simulink model "TV_2017"  (R2016a)
settings: Solver=FixedStepAuto  StartTime=0.0  StopTime=inf  FixedStep=0.001  RelTol=1e-3
PreLoadFcn:
  | TV_2017_parameters
values from neighbouring files (symbols this model uses):
  battery_voltage = single(530)    [HIL_parameters.m]    (also in HIL_parameters_2018.m; TV_2017_parameters.m; TV_2017_parameters_VD.m)
  car_params = Simulink_Car_params    [HIL_parameters.m]    (also in HIL_parameters_2018.m; TV_2017_parameters.m; TV_2017_parameters_VD.m)
  i_Diff = 16    [HIL_parameters.m]    (also in HIL_parameters_2018.m; TV_2017_parameters.m)
  Kp = 1    [HIL_parameters.m]    (also in HIL_parameters_2018.m; TV_2017_parameters.m; TV_2017_parameters_VD.m)
  motor_data = struct    [HIL_parameters.m]    (also in HIL_parameters_2018.m; TV_2017_parameters.m)
  powerLimitControl = Simulink_el    [HIL_parameters.m]    (also in HIL_parameters_2018.m; TV_2017_parameters.m; TV_2017_parameters_VD.m)
  settings = Simulink_Settings    [HIL_parameters.m]    (also in HIL_parameters_2018.m; TV_2017_parameters.m; TV_2017_parameters_VD.m)
  SpdC_BCC = 0    [HIL_parameters.m]    (also in HIL_parameters_2018.m; TV_2017_parameters.m; TV_2017_parameters_VD.m)
  Speed_Neg_sat = -21    [HIL_parameters.m]    (also in HIL_parameters_2018.m; TV_2017_parameters.m; TV_2017_parameters_VD.m)
  Speed_Pos_sat = 21    [HIL_parameters.m]    (also in HIL_parameters_2018.m; TV_2017_parameters.m; TV_2017_parameters_VD.m)
  SteeringAngleFL = [-23.80 -22.65 -21.50 -20.34 -19.18 -18.03 -16.86 -15.70 -14.53 -13.35 -12.18 -10.99 -9.80 -8.61 -7.40 -6.19 -4.97 -3.75 -2.51 -1.26 0 1.27 2.56 3.85 5.17 6.50 7.84 9.21 10.59 12.00 13.42 14.88 16.36 17.87 19.41 20.99 22.61 24.26 25.97 27.73 29.54]    [CarSetupAnalysis2018.m]    (also in HIL_parameters_2018.m; TV_2017_parameters.m; TV_2017_parameters_VD.m = [-24.129 -22.950 -21.772 -20.593 -19.413 -18.232 -17.050 -15)
  SteeringAngleFR = [-29.54 -27.73 -25.97 -24.26 -22.61 -20.99 -19.41 -17.87 -16.36 -14.88 -13.42 -12.00 -10.59 -9.21 -7.84 -6.50 -5.17 -3.85 -2.56 -1.27 0 1.26 2.51 3.75 4.97 6.19 7.40 8.61 9.80 10.99 12.18 13.35 14.53 15.70 16.86 18.03 19.18 20.34 21.50 22.65 23.80]    [CarSetupAnalysis2018.m]    (also in HIL_parameters_2018.m; TV_2017_parameters.m; TV_2017_parameters_VD.m = [-29.3050 -27.5340 -25.8140 -24.1410 -22.5110 -20.9180 -19.3)
  SteeringWhAngle = [-105 -99.75 -94.5 -89.25 -84 -78.75 -73.5 -68.25 -63 -57.75 -52.5 -47.25 -42 -36.75 -31.5 -26.25 -21.0 -15.75 -10.5 -5.25 0.0 5.25 10.50 15.75 21.00 26.25 31.50 36.75 42.00 47.25 52.50 57.75  63.00 68.25 73.50 78.75 84.00 89.25 94.50 99.75 105.00]    [TV_2017_parameters_VD.m]
  Tn_n = 0    [HIL_parameters.m]    (also in HIL_parameters_2018.m; TV_2017_parameters.m; TV_2017_parameters_VD.m)
  tractionControl = Simulink_tc    [HIL_parameters.m]    (also in HIL_parameters_2018.m; IterativeTractionControlTuning.m; TV_2017_parameters.m; TV_2017_parameters_VD.m)
  yawMomentGenerator = struct    [HIL_parameters.m]    (also in HIL_parameters_2018.m = Simulink_yawRate2; TV_2017_parameters.m = Simulink_yawRate2)
  yawRateControl = Simulink_yawRate    [HIL_parameters.m]    (also in HIL_parameters_2018.m; TV_2017_parameters.m; TV_2017_parameters_VD.m)
undefined symbols (not defined in the file or in its folder): DiscIntNeverNeededParam, magnitude, speedEstimation, TC_Decr_Gas, TC_Derivative, TC_Incr_Gas, TC_On, TC_Relay_Off, TC_Relay_On
libraries: CarMaker4SL x350, simulink_extras x63, simulink x37, dspfdesign x2
(part 5 of 14)

== system TV_2017/CarMaker/Estimations/createStateBus ==
  mean_wheel_angle : Inport
  mean_wheel_speed : Inport  Port=2
  Fx : Inport  Port=3
  sensors : Inport  Port=4
  Fz_est : Inport  Port=5
  whl_speed_cog : Inport  Port=6
  SR : Inport  Port=7
  frictionCoefficient : Inport  Port=8
  SA : Inport  Port=9
  v_x : Inport  Port=10
  v_y : Inport  Port=11
  slip : Inport  Port=12
  Bus Creator1 : BusCreator  Inputs=52  OutDataTypeStr=Bus: States  NonVirtualBus=on
      settings: InheritFromInputs=off
  Bus Selector{,2..6} (6 alike) : BusSelector  OutputSignals=FL,FR,RL,RR
  Bus Selector1 : BusSelector  OutputSignals=Input_throttle,Input_brake,KERS_pos,yawRate,yawRate_der,ax,ay,RPM_FL,RPM_FR,RPM_RL,RPM_RR,power,DC_voltage,AMK_motor_temp_FL,AMK_motor_temp_FR,AMK_motor_temp_RL,AMK_motor_temp_RR,AMK_inverter_temp_FL,AMK_inverter_temp_FR,AMK_inverter_temp_RL,AMK_inverter_temp_RR,steering_wheel_angle,steering_wheel_speed
  states : Outport
  wires:
  sensors/1 -> Bus Selector1/1
  Fz_est/1 -> Bus Selector/1
  whl_speed_cog/1 -> Bus Selector2/1
  Fx/1 -> Bus Selector3/1
  SR/1 -> Bus Selector4/1
  Bus Selector1/9 -> Bus Creator1/9  "<RPM_FR>"
  Bus Selector1/8 -> Bus Creator1/8  "<RPM_FL>"
  Bus Selector1/10 -> Bus Creator1/10  "<RPM_RL>"
  Bus Selector1/7 -> Bus Creator1/7  "<ay>"
  Bus Selector1/11 -> Bus Creator1/11  "<RPM_RR>"
  Bus Selector1/6 -> Bus Creator1/6  "<ax>"
  Bus Selector1/12 -> Bus Creator1/12  "<power>"
  Bus Selector1/5 -> Bus Creator1/5  "<yawRate_der>"
  Bus Selector1/13 -> Bus Creator1/13  "<DC_voltage>"
  Bus Selector1/4 -> Bus Creator1/4  "<yawRate>"
  Bus Selector1/3 -> Bus Creator1/3  "<KERS_pos>"
  Bus Selector1/2 -> Bus Creator1/2  "<Input_brake>"
  Bus Selector1/1 -> Bus Creator1/1  "<Input_throttle>"
  mean_wheel_angle/1 -> Bus Creator1/24
  mean_wheel_speed/1 -> Bus Creator1/25
  v_x/1 -> Bus Creator1/26
  v_y/1 -> Bus Creator1/27
  Bus Selector/1 -> Bus Creator1/32  "<FL>"
  Bus Selector/2 -> Bus Creator1/33  "<FR>"
  Bus Selector/3 -> Bus Creator1/34  "<RL>"
  Bus Selector/4 -> Bus Creator1/35  "<RR>"
  Bus Selector2/1 -> Bus Creator1/36  "<FL>"
  Bus Selector2/2 -> Bus Creator1/37  "<FR>"
  Bus Selector2/3 -> Bus Creator1/38  "<RL>"
  Bus Selector2/4 -> Bus Creator1/39  "<RR>"
  Bus Selector4/1 -> Bus Creator1/40  "<FL>"
  Bus Selector4/2 -> Bus Creator1/41  "<FR>"
  Bus Selector4/3 -> Bus Creator1/42  "<RL>"
  Bus Selector4/4 -> Bus Creator1/43  "<RR>"
  Bus Selector3/1 -> Bus Creator1/28  "<FL>"
  Bus Selector3/2 -> Bus Creator1/29  "<FR>"
  Bus Selector3/3 -> Bus Creator1/30  "<RL>"
  Bus Selector3/4 -> Bus Creator1/31  "<RR>"
  frictionCoefficient/1 -> Bus Creator1/52
  Bus Selector1/14 -> Bus Creator1/14  "<AMK_motor_temp_FL>"
  Bus Selector1/15 -> Bus Creator1/15  "<AMK_motor_temp_FR>"
  Bus Selector1/16 -> Bus Creator1/16  "<AMK_motor_temp_RL>"
  Bus Selector1/17 -> Bus Creator1/17  "<AMK_motor_temp_RR>"
  Bus Selector1/18 -> Bus Creator1/18  "<AMK_inverter_temp_FL>"
  Bus Selector1/19 -> Bus Creator1/19  "<AMK_inverter_temp_FR>"
  Bus Selector1/20 -> Bus Creator1/20  "<AMK_inverter_temp_RL>"
  Bus Selector1/21 -> Bus Creator1/21  "<AMK_inverter_temp_RR>"
  SA/1 -> Bus Selector5/1
  Bus Selector5/1 -> Bus Creator1/44  "<FL>"
  Bus Selector5/2 -> Bus Creator1/45  "<FR>"
  Bus Selector5/3 -> Bus Creator1/46  "<RL>"
  Bus Selector5/4 -> Bus Creator1/47  "<RR>"
  Bus Creator1/1 -> states/1
  Bus Selector1/22 -> Bus Creator1/22  "<steering_wheel_angle>"
  Bus Selector1/23 -> Bus Creator1/23  "<steering_wheel_speed>"
  slip/1 -> Bus Selector6/1
  Bus Selector6/1 -> Bus Creator1/48  "<FL>"
  Bus Selector6/2 -> Bus Creator1/49  "<FR>"
  Bus Selector6/3 -> Bus Creator1/50  "<RL>"
  Bus Selector6/4 -> Bus Creator1/51  "<RR>"

== system TV_2017/CarMaker/Estimations/friction_estimation ==
  Fx : Inport
  SR : Inport  Port=2
  Fz : Inport  Port=3
  estimateFrictionCoefficient : MATLAB Function  TreatAsAtomicUnit=on
  mu : Outport
  mu_estimate : Outport  Port=2
  mu_individual : Outport  Port=3
  normLongTireForce : Outport  Port=4
  wires:
  Fx/1 -> estimateFrictionCoefficient/1(Fx)
  Fz/1 -> estimateFrictionCoefficient/2(Fz)
  SR/1 -> estimateFrictionCoefficient/3(SR)
  estimateFrictionCoefficient/1(mu) -> mu/1
  estimateFrictionCoefficient/3(normLongTireForce) -> normLongTireForce/1
  estimateFrictionCoefficient/2(mu_estimate) -> mu_estimate/1

== system TV_2017/CarMaker/Estimations/selectVelocity ==
  v_est_x : Inport
  sensors : Inport  Port=2
  Bus Selector : BusSelector  OutputSignals=V_x_INS,V_x_optical
  Bus Selector1 : BusSelector  OutputSignals=V_y_INS,V_y_optical
  Constant1 : Constant  Value=settings.select_velocity_vx
  Constant2 : Constant  Value=settings.select_velocity_vy
  Index Vector : MultiPortSwitch
  Index Vector1 : MultiPortSwitch  DataPortOrder=Specify indices  Inputs=2  DataPortIndices={2,3}
  v_x : Outport
  v_y : Outport  Port=2
  wires:
  Constant1/1 -> Index Vector/1
  v_est_x/1 -> Index Vector/2
  sensors/1 -> Bus Selector1/1, Bus Selector/1
  Bus Selector/1 -> Index Vector/3  "<V_x_INS>"
  Bus Selector/2 -> Index Vector/4  "<V_x_optical>"
  Index Vector/1 -> v_x/1
  Constant2/1 -> Index Vector1/1
  Bus Selector1/1 -> Index Vector1/2  "<V_y_INS>"
  Bus Selector1/2 -> Index Vector1/3  "<V_y_optical>"
  Index Vector1/1 -> v_y/1

== system TV_2017/CarMaker/IPG Vehicle3/Brake ==
  note: When replacing the entire braking system,
      | be sure to add '-disablebrake' to the command line arguments
      | in the CarMaker Model Configuration block.
  note: <Your model here>
  Sync_In : Inport
  Brake.IF.In : Inport  Port=2
  VhclCtrl.Brake : Inport  Port=3
  Brake : S-Function  FunctionName=CM_Sfun  Parameters='Brake'  SFunctionDeploymentMode=off  EnableBusSupport=off
  BrakeUpd : S-Function  FunctionName=CM_Sfun  Parameters='BrakeUpd'  SFunctionDeploymentMode=off  EnableBusSupport=off
  BusCreator1 : BusCreator  Inputs=16
  CreateBus Vhcl.Wheel.PT : Subsystem
  Demux : Demux  Outputs=16
  Sync_Out : Outport
  Vhcl.Wheel.PT : Outport  Port=2
  wires:
  Demux/16 -> BusCreator1/16  "Brake IF Trq_DriveSrc_trg d3"
  Demux/15 -> BusCreator1/15  "Brake IF Trq_DriveSrc_trg d2"
  Demux/14 -> BusCreator1/14  "Brake IF Trq_DriveSrc_trg d1"
  Demux/13 -> BusCreator1/13  "Brake IF Trq_DriveSrc_trg d0"
  Demux/12 -> BusCreator1/12  "Brake IF Trq_Reg_trg RR"
  Demux/11 -> BusCreator1/11  "Brake IF Trq_Reg_trg RL"
  Demux/10 -> BusCreator1/10  "Brake IF Trq_Reg_trg FR"
  Demux/9 -> BusCreator1/9  "Brake IF Trq_Reg_trg FL"
  Demux/8 -> BusCreator1/8  "Brake IF Trq_PB RR"
  Demux/7 -> BusCreator1/7  "Brake IF Trq_PB RL"
  Demux/6 -> BusCreator1/6  "Brake IF Trq_PB FR"
  Demux/5 -> BusCreator1/5  "Brake IF Trq_PB FL"
  Demux/4 -> BusCreator1/4  "Brake IF Trq_WB RR"
  Demux/3 -> BusCreator1/3  "Brake IF Trq_WB RL"
  Demux/2 -> BusCreator1/2  "Brake IF Trq_WB FR"
  Demux/1 -> BusCreator1/1  "Brake IF Trq_WB FL"
  Brake/2 -> Demux/1
  BusCreator1/1 -> BrakeUpd/2
  BrakeUpd/1 -> Sync_Out/1
  Brake/1 -> BrakeUpd/1  "Sync"
  Brake.IF.In/1 -> Brake/2
  VhclCtrl.Brake/1 -> Brake/3
  Sync_In/1 -> Brake/1
  BrakeUpd/2 -> CreateBus Vhcl.Wheel.PT/1(In)
  CreateBus Vhcl.Wheel.PT/1(Out) -> Vhcl.Wheel.PT/1

== system TV_2017/CarMaker/IPG Vehicle3/CarAndTrailer ==
  Sync_In : Inport
  VhclCtrl.Steering : Inport  Port=2
  Vhcl.Wheel.In : Inport  Port=3
  Vhcl.Misc : Inport  Port=4
  CarAndTrailerUpd : Subsystem
  Forces : Subsystem
  Ground : Ground
  Kinematics : Subsystem
  Kinetics : Subsystem
  Steering : Subsystem
  Terminator : Terminator
  Terminator1 : Terminator
  Trailer : Subsystem
  Sync_Out : Outport
  Brake.IF.In : Outport  Port=2
  wires:
  Trailer/9(Car.Hitch.FrcTrq) -> CarAndTrailerUpd/9(Car.Hitch.FrcTrq)
  Trailer/8(Vhcl.Wheel.RR) -> CarAndTrailerUpd/8(Vhcl.Wheel.RR)
  Trailer/7(Vhcl.Wheel.RL) -> CarAndTrailerUpd/7(Vhcl.Wheel.RL)
  Trailer/6(Vhcl.Wheel.FR) -> CarAndTrailerUpd/6(Vhcl.Wheel.FR)
  Trailer/5(Vhcl.Wheel.FL) -> CarAndTrailerUpd/5(Vhcl.Wheel.FL)
  Trailer/4(Vhcl.PoI) -> CarAndTrailerUpd/4(Vhcl.PoI)
  Trailer/3(Vhcl.Motion) -> CarAndTrailerUpd/3(Vhcl.Motion)
  Trailer/2(Vhcl.Steering) -> CarAndTrailerUpd/2(Vhcl.Steering)
  Trailer/1(Sync_Out) -> CarAndTrailerUpd/1(Sync_In)
  CarAndTrailerUpd/2(Brake.IF.In) -> Brake.IF.In/1
  CarAndTrailerUpd/1(Sync_Out) -> Sync_Out/1
  Vhcl.Misc/1 -> Terminator1/1
  Vhcl.Wheel.In/1 -> Terminator/1
  Kinetics/6(WheelCarrier.Misc) -> Trailer/6(WheelCarrier.Misc)
  Kinetics/5(Car.Trq_T2W) -> Trailer/5(Car.Trq_T2W)
  Steering/2(Steer.IF) -> Kinematics/2(Steer.IF)
  Kinetics/4(Car.Fr1) -> Trailer/4(Car.Fr1)
  Kinetics/3(Car.Hitch) -> Trailer/3(Car.Hitch)
  Kinetics/2(Trailer.Load) -> Trailer/2(Trailer.Load)
  VhclCtrl.Steering/1 -> Steering/2(VhclCtrl.Steering)
  Sync_In/1 -> Steering/1(Sync_In)
  Steering/1(Sync_Out) -> Kinematics/1(Sync_In)
  Kinetics/1(Sync_Out) -> Trailer/1(Sync_In)
  Ground/1 -> CarAndTrailerUpd/10(Vhcl.Fr1A)
  Forces/11(FStabi) -> Kinetics/11(FStabi)
  Forces/10(FDamp) -> Kinetics/10(FDamp)
  Forces/9(FSpring) -> Kinetics/9(FSpring)
  Forces/8(TireRR_Out) -> Kinetics/8(TireRR.Out)
  Forces/7(TireRL_Out) -> Kinetics/7(TireRL.Out)
  Forces/6(TireFR_Out) -> Kinetics/6(TireFR.Out)
  Forces/5(TireFL_Out) -> Kinetics/5(TireFL.Out)
  Forces/4(Car.Load) -> Kinetics/4(Car.Load)
  Forces/2(Car.Virtual) -> Kinetics/2(Car.Virtual)
  Kinematics/6(lSpring) -> Forces/6(lSpring)
  Kinematics/7(vDamp) -> Forces/7(vDamp)
  Forces/3(Car.Aero) -> Kinetics/3(Car.Aero)
  Forces/1(Sync_Out) -> Kinetics/1(Sync_In)
  Kinematics/5(TireRR_In) -> Forces/5(TireRR_In)
  Kinematics/4(TireRL_In) -> Forces/4(TireRL_In)
  Kinematics/3(TireFR_In) -> Forces/3(TireFR_In)
  Kinematics/2(TireFL_In) -> Forces/2(TireFL_In)
  Kinematics/1(Sync_Out) -> Forces/1(Sync_In)
  Kinematics/8(lStabi) -> Forces/8(lStabi)
  Forces/12(FBuf) -> Kinetics/12(FBuf)
  Kinematics/9(lBuf) -> Forces/9(lBuf)

== system TV_2017/CarMaker/IPG Vehicle3/PowerTrain ==
  note: When replacing the entire powertrain,
      | be sure to add '-disablepowertrain' to the command line arguments
      | in the CarMaker Model Configuration block.
  note: <Your model here>
  Sync_In : Inport
  Vhcl.Wheel.PT : Inport  Port=2
  VhclCtrl.PT : Inport  Port=3
  BusCreator1 : BusCreator  Inputs=42
  Demux1 : Demux  Outputs=42
  Electric Powertrain : Subsystem
  PowerTrain : S-Function  FunctionName=CM_Sfun  Parameters='PowerTrain'  SFunctionDeploymentMode=off  EnableBusSupport=off
  PowerTrainUpd : S-Function  FunctionName=CM_Sfun  Parameters='PowerTrainUpd'  SFunctionDeploymentMode=off  EnableBusSupport=off
  Saturation : Saturate  Commented=on  UpperLimit=2*pi*16000/60  LowerLimit=2*pi*100/60
  Terminator : Terminator
  Terminator1 : Terminator
  Sync_Out : Outport
  wires:
  BusCreator1/1 -> PowerTrainUpd/2
  Demux1/42 -> BusCreator1/42  "PT IF WRR Trq_BrakeReg_max"
  Demux1/41 -> BusCreator1/41  "PT IF WRR Trq_BrakeReg"
  Demux1/40 -> BusCreator1/40  "PT IF WRR Trq_Supp2WC"
  Demux1/38 -> BusCreator1/38  "PT IF WRR Trq_B2W"
  Demux1/37 -> BusCreator1/37  "PT IF WRR rotv"
  Demux1/36 -> BusCreator1/36  "PT IF WRR rot"
  Demux1/35 -> BusCreator1/35  "PT IF WRL Trq_BrakeReg_max"
  Demux1/34 -> BusCreator1/34  "PT IF WRL Trq_BrakeReg"
  Demux1/33 -> BusCreator1/33  "PT IF WRL Trq_Supp2WC"
  Demux1/31 -> BusCreator1/31  "PT IF WRL Trq_B2W"
  Demux1/30 -> BusCreator1/30  "PT IF WRL rotv"
  Demux1/29 -> BusCreator1/29  "PT IF WRL rot"
  Demux1/28 -> BusCreator1/28  "PT IF WFR Trq_BrakeReg_max"
  Demux1/27 -> BusCreator1/27  "PT IF WFR Trq_BrakeReg"
  Demux1/26 -> BusCreator1/26  "PT IF WFR Trq_Supp2WC"
  Demux1/24 -> BusCreator1/24  "PT IF WFR Trq_B2W"
  Demux1/23 -> BusCreator1/23  "PT IF WFR rotv"
  Demux1/22 -> BusCreator1/22  "PT IF WFR rot"
  Demux1/21 -> BusCreator1/21  "PT IF WFL Trq_BrakeReg_max"
  Demux1/20 -> BusCreator1/20  "PT IF WFL Trq_BrakeReg"
  Demux1/19 -> BusCreator1/19  "PT IF WFL Trq_Supp2WC"
  Demux1/17 -> BusCreator1/17  "PT IF WFL Trq_B2W"
  Demux1/16 -> BusCreator1/16  "PT IF WFL rotv"
  Demux1/15 -> BusCreator1/15  "PT IF WFL rot"
  Demux1/14 -> BusCreator1/14  "PT IF DL_iDiff_mean"
  Demux1/13 -> BusCreator1/13  "PT IF Trq_Supp2BdyEng y"
  Demux1/12 -> BusCreator1/12  "PT IF Trq_Supp2BdyEng x"
  Demux1/11 -> BusCreator1/11  "PT IF Trq_Supp2Bdy1B z"
  Demux1/10 -> BusCreator1/10  "PT IF Trq_Supp2Bdy1B y"
  Demux1/9 -> BusCreator1/9  "PT IF Trq_Supp2Bdy1B x"
  Demux1/8 -> BusCreator1/8  "PT IF Trq_Supp2Bdy1 z"
  Demux1/7 -> BusCreator1/7  "PT IF Trq_Supp2Bdy1 y"
  Demux1/6 -> BusCreator1/6  "PT IF Trq_Supp2Bdy1 x"
  Demux1/4 -> BusCreator1/4  "PT IF GearNo"
  Demux1/3 -> BusCreator1/3  "PT IF OperationError"
  Demux1/1 -> BusCreator1/1  "PT IF Ignition"
  Sync_In/1 -> PowerTrain/1
  PowerTrain/2 -> Demux1/1
  PowerTrainUpd/1 -> Sync_Out/1
  PowerTrain/1 -> PowerTrainUpd/1  "Sync"
  VhclCtrl.PT/1 -> PowerTrain/3
  Vhcl.Wheel.PT/1 -> PowerTrain/2
  Demux1/2 -> Terminator/1  "PT IF OperationState"
  Demux1/5 -> Terminator1/1  "PT IF Engine_rotv"
  Electric Powertrain/1(PT.OperationState1) -> BusCreator1/2
  Electric Powertrain/2(PT.Engine.rotv1) -> BusCreator1/5
  Electric Powertrain/3(T_FL) -> BusCreator1/18
  Electric Powertrain/4(T_FR) -> BusCreator1/25
  Electric Powertrain/5(T_RL) -> BusCreator1/32
  Electric Powertrain/6(T_RR) -> BusCreator1/39

== system TV_2017/CarMaker/VehicleControl3/CreateBus Vhcl.Misc ==
  In1 : Inport
  BusCreator : BusCreator  Inputs=11
  Demux : Demux  Outputs=11
  Out1 : Outport
  wires:
  Demux/11 -> BusCreator/11  "Vhcl Wind_vel_0 z"
  Demux/10 -> BusCreator/10  "Vhcl Wind_vel_0 y"
  Demux/9 -> BusCreator/9  "Vhcl Wind_vel_0 x"
  Demux/8 -> BusCreator/8  "Vhcl Trq_DL2BdyEng y"
  Demux/7 -> BusCreator/7  "Vhcl Trq_DL2BdyEng x"
  Demux/6 -> BusCreator/6  "Vhcl Trq_DL2Bdy1B z"
  Demux/5 -> BusCreator/5  "Vhcl Trq_DL2Bdy1B y"
  Demux/4 -> BusCreator/4  "Vhcl Trq_DL2Bdy1B x"
  Demux/3 -> BusCreator/3  "Vhcl Trq_DL2Bdy1 z"
  Demux/2 -> BusCreator/2  "Vhcl Trq_DL2Bdy1 y"
  Demux/1 -> BusCreator/1  "Vhcl Trq_DL2Bdy1 x"
  In1/1 -> Demux/1
  BusCreator/1 -> Out1/1

== system TV_2017/CarMaker/VehicleControl3/CreateBus Vhcl.Wheel.In ==
  In1 : Inport
  Bus Creator1 : BusCreator  Inputs=12
  Demux1 : Demux  Outputs=12
  Out1 : Outport
  wires:
  Demux1/12 -> Bus Creator1/12  "Vhcl Wheel RR rotv"
  Demux1/11 -> Bus Creator1/11  "Vhcl Wheel RR Trq_DL2WC"
  Demux1/10 -> Bus Creator1/10  "Vhcl Wheel RR Trq_B2WC"
  Demux1/9 -> Bus Creator1/9  "Vhcl Wheel RL rotv"
  Demux1/8 -> Bus Creator1/8  "Vhcl Wheel RL Trq_DL2WC"
  Demux1/7 -> Bus Creator1/7  "Vhcl Wheel RL Trq_B2WC"
  Demux1/6 -> Bus Creator1/6  "Vhcl Wheel FR rotv"
  Demux1/5 -> Bus Creator1/5  "Vhcl Wheel FR Trq_DL2WC"
  Demux1/4 -> Bus Creator1/4  "Vhcl Wheel FR Trq_B2WC"
  Demux1/3 -> Bus Creator1/3  "Vhcl Wheel FL rotv"
  In1/1 -> Demux1/1
  Bus Creator1/1 -> Out1/1
  Demux1/2 -> Bus Creator1/2  "Vhcl Wheel FL Trq_DL2WC"
  Demux1/1 -> Bus Creator1/1  "Vhcl Wheel FL Trq_B2WC"

== system TV_2017/CarMaker/VehicleControl3/CreateBus VhclCtrl ==
  In : Inport
  BusCreator : BusCreator  Inputs=29
  Demux : Demux  Outputs=29
  Out : Outport
  wires:
  In/1 -> Demux/1
  BusCreator/1 -> Out/1
  Demux/1 -> BusCreator/1  "VhclCtrl SST"
  Demux/2 -> BusCreator/2  "VhclCtrl Key"
  Demux/3 -> BusCreator/3  "VhclCtrl UserSignal0"
  Demux/4 -> BusCreator/4  "VhclCtrl UserSignal1"
  Demux/5 -> BusCreator/5  "VhclCtrl UserSignal2"
  Demux/6 -> BusCreator/6  "VhclCtrl UserSignal3"
  Demux/7 -> BusCreator/7  "VhclCtrl UserSignal4"
  Demux/8 -> BusCreator/8  "VhclCtrl GearNo"
  Demux/9 -> BusCreator/9  "VhclCtrl SelectorCtrl"
  Demux/10 -> BusCreator/10  "VhclCtrl Brake"
  Demux/11 -> BusCreator/11  "VhclCtrl BrakePark"
  Demux/12 -> BusCreator/12  "VhclCtrl Clutch"
  Demux/13 -> BusCreator/13  "VhclCtrl Gas"
  Demux/14 -> BusCreator/14  "VhclCtrl Steering Ang"
  Demux/15 -> BusCreator/15  "VhclCtrl Steering AngVel"
  Demux/16 -> BusCreator/16  "VhclCtrl Steering AngAcc"
  Demux/17 -> BusCreator/17  "VhclCtrl Steering Trq"
  Demux/18 -> BusCreator/18  "VhclCtrl Lights LowBeam"
  Demux/19 -> BusCreator/19  "VhclCtrl Lights HighBeam"
  Demux/20 -> BusCreator/20  "VhclCtrl Lights Daytime"
  Demux/21 -> BusCreator/21  "VhclCtrl Lights ParkL"
  Demux/22 -> BusCreator/22  "VhclCtrl Lights ParkR"
  Demux/23 -> BusCreator/23  "VhclCtrl Lights IndL"
  Demux/24 -> BusCreator/24  "VhclCtrl Lights IndR"
  Demux/25 -> BusCreator/25  "VhclCtrl Lights FogFrontL"
  Demux/26 -> BusCreator/26  "VhclCtrl Lights FogFrontR"
  Demux/27 -> BusCreator/27  "VhclCtrl Lights FogRear"
  Demux/28 -> BusCreator/28  "VhclCtrl Lights Brake"
  Demux/29 -> BusCreator/29  "VhclCtrl Lights Reverse"

== system TV_2017/CarMaker/VehicleControl3/CreateBus VhclCtrl.PT ==
  In1 : Inport
  BusCreator1 : BusCreator  Inputs=12
  Demux1 : Demux  Outputs=12
  Out1 : Outport
  wires:
  Demux1/12 -> BusCreator1/12  "VhclCtrl Brake"
  Demux1/11 -> BusCreator1/11  "VhclCtrl Gas"
  Demux1/10 -> BusCreator1/10  "VhclCtrl Clutch"
  Demux1/9 -> BusCreator1/9  "VhclCtrl SelectorCtrl"
  Demux1/8 -> BusCreator1/8  "VhclCtrl GearNo"
  Demux1/7 -> BusCreator1/7  "VhclCtrl UserSignal4"
  Demux1/6 -> BusCreator1/6  "VhclCtrl UserSignal3"
  Demux1/5 -> BusCreator1/5  "VhclCtrl UserSignal2"
  Demux1/4 -> BusCreator1/4  "VhclCtrl UserSignal1"
  Demux1/3 -> BusCreator1/3  "VhclCtrl UserSignal0"
  Demux1/2 -> BusCreator1/2  "VhclCtrl Key"
  Demux1/1 -> BusCreator1/1  "VhclCtrl SST"
  In1/1 -> Demux1/1
  BusCreator1/1 -> Out1/1

== system TV_2017/CarMaker/VehicleControl3/CreateBus VhclCtrl.Steering ==
  In1 : Inport
  Bus Creator : BusCreator  Inputs=5
  Demux : Demux  Outputs=5
  Out1 : Outport
  wires:
  In1/1 -> Demux/1
  Bus Creator/1 -> Out1/1
  Demux/1 -> Bus Creator/1  "VhclCtrl Steering Ang"
  Demux/5 -> Bus Creator/5  "VhclCtrl Steering SteerByTrq"
  Demux/3 -> Bus Creator/3  "VhclCtrl Steering AngAcc"
  Demux/2 -> Bus Creator/2  "VhclCtrl Steering AngVel"
  Demux/4 -> Bus Creator/4  "VhclCtrl Steering Trq"

== system TV_2017/CarMaker/Control_System /Power Limit Torque Reduction Controller 2018/Motorestimates ==
  states : Inport
  Ti_lim : Inport  Port=2
  Scope : Scope  NumInputPorts=4
  Scope1 : Scope  NumInputPorts=4
  extractPower2 : MATLAB Function  TreatAsAtomicUnit=on
  motor efficiency table based on RPM and torque{,1..3} (4 alike) : Lookup_n-D  BreakpointsForDimension1=single([1.3,2.7,5.4,7.9,10.4,12.5,14.4,16.0,17.4,18.5,19.6]);  BreakpointsForDimension2=single([500,1000,2000,3000,4000,6000,10000,12000,15000,19000]);  Table=single(reshape([0.6437000036239624,0.5799999833106995,0.44999998807907104,0.3499999940395355,0.28999999165534973,0.23999999463558197,0.20000000298023224,0.17000000178813934,0.14000000059604645,0.12999999523162842,0.10999999940395355,0.7099999785423279,0.699999988079071,0.6100000143051148,0.5099999904632568,0.4399999976158142,0.3799999952316284,0.33000001311302185,0.28999999165534973,0.25,0.2199999988079071,0.20000000298023224,0.7300000190734863,0.7699999809265137,0.7300000190734863,0.6700000166893005,0.6100000143051148,0.550000011920929,0.5,0.44999998807907104,0.4000000059604645,0.36000001430511475,0.33000001311302185,0.7400000095367432,0.800000011920929,0.7900000214576721,0.7400000095367432,0.6899999976158142,0.6399999856948853,0.5899999737739563,0.5400000214576721,0.5,0.46000000834465027,0.41999998688697815,0.75,0.8199999928474426,0.8199999928474426,0.7799999713897705,0.7400000095367432,0.699999988079071,0.6600000262260437,0.6100000143051148,0.5699999928474426,0.5299999713897705,0.49000000953674316,0.7599999904632568,0.8399999737739563,0.8500000238418579,0.8299999833106995,0.800000011920929,0.7699999809265137,0.7400000095367432,0.699999988079071,0.6600000262260437,0.6200000047683716,0.5899999737739563,0.7699999809265137,0.8500000238418579,0.8799999952316284,0.8700000047683716,0.8600000143051148,0.8399999737739563,0.8100000023841858,0.7799999713897705,0.7599999904632568,0.7200000286102295,0.699999988079071,0.7699999809265137,0.8500000238418579,0.8899999856948853,0.8799999952316284,0.8700000047683716,0.8500000238418579,0.8299999833106995,0.8100000023841858,0.7799999713897705,0.7599999904632568,0.7300000190734863,0.7699999809265137,0.8600000143051148,0.8999999761581421,0.8999999761581421,0.8899999856948853,0.8700000047683716,0.8500000238418579,0.8299999833106995,0.8100000023841858,0.7900000214576721,0.6700000166893005,0.7799999713897705,0.8600000143051148,0.8999999761581421,0.9100000262260437,0.8999999761581421,0.8899999856948853,0.8700000047683716,0.8600000143051148,0.8299999833106995,0.7699999809265137,0.699999988079071],11,10));  ExtrapMethod=Clip  UseLastTableValue=on  InternalRulePriority=Speed  RndMeth=Simplest  InputSameDT=on
  Eff_FL : Outport
  Eff_FR : Outport  Port=2
  Eff_RL : Outport  Port=3
  Eff_RR : Outport  Port=4
  wires:
  extractPower2/4(RPM_FR) -> motor efficiency table based on RPM and torque1/2
  motor efficiency table based on RPM and torque/1 -> Scope1/1, Eff_FL/1
  motor efficiency table based on RPM and torque2/1 -> Eff_RL/1
  motor efficiency table based on RPM and torque3/1 -> Eff_RR/1
  Ti_lim/1 -> extractPower2/2(Ti_lim)
  states/1 -> extractPower2/1(states)
  motor efficiency table based on RPM and torque1/1 -> Eff_FR/1
  extractPower2/2(RPM_FL) -> motor efficiency table based on RPM and torque/2
  extractPower2/6(RPM_RL) -> motor efficiency table based on RPM and torque2/2
  extractPower2/1(T_FL) -> Scope/1, motor efficiency table based on RPM and torque/1
  extractPower2/8(RPM_RR) -> motor efficiency table based on RPM and torque3/2
  extractPower2/5(T_RL) -> motor efficiency table based on RPM and torque2/1
  extractPower2/3(T_FR) -> motor efficiency table based on RPM and torque1/1
  extractPower2/7(T_RR) -> motor efficiency table based on RPM and torque3/1

== system TV_2017/CarMaker/Control_System /Power Limit Torque Reduction Controller 2018/Old powerlimiting  ==
  ti_lim : Inport
  states : Inport  Port=2
  Abs : Abs
  Add : Sum
  Bus Creator : BusCreator  Inputs=4  OutDataTypeStr=Bus: Ti_lim  NonVirtualBus=on
      settings: InheritFromInputs=off
  Bus Selector : BusSelector  OutputSignals=FL,FR,RL,RR
  Discrete PI controller : simulink/Continuous/PID Controller  Controller=PI  TimeDomain=Discrete-time  SampleTime=-1  IntegratorMethod=Forward Euler  FilterMethod=Forward Euler  Form=Parallel  UseFilter=on  ControllerParametersSource=internal  P=powerLimitControl.Kp  I=powerLimitControl.Ki  D=0  N=100  InitialConditionSource=internal  InitialConditionForIntegrator=0  InitialConditionForFilter=0  ExternalReset=none  LimitOutput=on  UpperSaturationLimit=powerLimitControl.upper_sat_limit  LowerSaturationLimit=powerLimitControl.lower_sat_limit  LinearizeAsGain=off  AntiWindupMode=clamping  Kb=settings.Kb_EL;  TrackingMode=off  Kt=1  PParamMin=[]  PParamMax=[]  IParamMin=[]  IParamMax=[]  DParamMin=[]  DParamMax=[]  NParamMin=[]  NParamMax=[]  KbParamMin=[]  KbParamMax=[]  KtParamMin=[]  KtParamMax=[]  POutMin=[]  POutMax=[]  IOutMin=[]  IOutMax=[]  DOutMin=[]  DOutMax=[]  NOutMin=[]  NOutMax=[]  KbOutMin=[]  KbOutMax=[]  KtOutMin=[]  KtOutMax=[]  IntegratorOutMin=[]  IntegratorOutMax=[]  FilterOutMin=[]  FilterOutMax=[]  SumOutMin=[]  SumOutMax=[]  SumI1OutMin=[]  SumI1OutMax=[]  SumI2OutMin=[]  SumI2OutMax=[]  SumI3OutMin=[]  SumI3OutMax=[]  SumDOutMin=[]  SumDOutMax=[]  SaturationOutMin=[]  SaturationOutMax=[]  IntegratorContinuousStateAttributes=''  IntegratorStateMustResolveToSignalObject=off  IntegratorRTWStateStorageClass=Auto  FilterContinuousStateAttributes=''  FilterStateMustResolveToSignalObject=off  FilterRTWStateStorageClass=Auto  DifferentiatorICPrevScaledInput=0  DifferentiatorOutMin=[]  DifferentiatorOutMax=[]
  Negative Power limit : Constant  Value=powerLimitControl.negative_power_limit
  "Positive Power limit " : Constant  Value=powerLimitControl.positive_power_limit
  Product{1..3,5} (4 alike) : Product
  Saturation : Saturate  UpperLimit=1  LowerLimit=0
  Scope : Scope
  Sum : Sum  Inputs=|+-
  Switch : Switch  Criteria=u2 > Threshold
  Switch1 : Switch  Threshold=1
  constant : Constant  Value=single(1)
  constant1 : Constant  Value=powerLimitControl.enable
  constant2 : Constant  Value=single(1)
  exact power : Scope
  extractPower1 : MATLAB Function  TreatAsAtomicUnit=on
  post red fac : Scope
  pre fact : Scope
  "ti_lim " : Outport
  wires:
  Bus Selector/4 -> Product3/2, pre fact/1  "<RR>"
  Bus Selector/1 -> Product5/2  "<FL>"
  Switch1/1 -> Saturation/1
  Bus Selector/2 -> Product2/2  "<FR>"
  Product1/1 -> Bus Creator/3  "RL"
  Discrete PI controller/1 -> Add/2
  Switch/1 -> Sum/1
  Bus Selector/3 -> Product1/2  "<RL>"
  ti_lim/1 -> Bus Selector/1
  Bus Creator/1 -> "ti_lim "/1
  Negative Power limit/1 -> Switch/3
  constant/1 -> Add/1
  Saturation/1 -> Product2/1, Product5/1, Product1/1, Product3/1
  Abs/1 -> Sum/2
  Product2/1 -> Bus Creator/2  "FR"
  "Positive Power limit "/1 -> Switch/1
  Product3/1 -> post red fac/1, Bus Creator/4  "RR"
  extractPower1/1(power) -> Switch/2, exact power/1, Abs/1
  Sum/1 -> Discrete PI controller/1
  states/1 -> extractPower1/1(states)
  Product5/1 -> Bus Creator/1  "FL"
  constant1/1 -> Scope/1, Switch1/2
  constant2/1 -> Switch1/3
  Add/1 -> Switch1/1

== system TV_2017/CarMaker/Control_System /Slip Rate Control /SMC Traction Control ==
  note: Tc ouput is either an increase or decrease in torque .
  states : Inport
  Ti_ref : Inport  Port=2
  T_requested : Inport  Port=3
  Bus Selector : BusSelector  OutputSignals=FL,FR,RL,RR
  Constant : Constant  Value=tractionControl.Kp
  Constant1 : Constant  Value=tractionControl.Ki
  Constant2 : Constant  Value=tractionControl.Slip_ratio_ref
  Gain : Gain  Gain=single(3.6)
  Gain2 : Gain  Gain=single(3.6)
  Ki Loopup : Lookup_n-D  NumberOfTableDimensions=1  BreakpointsForDimension1=[0 5 10]  Table="[tractionControl.Ki_start tractionControl.Ki_middle  tractionControl.Ki_end]*tractionControl.Ki_scaling"  ExtrapMethod=Clip  UseLastTableValue=on  InternalRulePriority=Speed  RndMeth=Simplest  InputSameDT=on
  Kp Lookup : Lookup_n-D  NumberOfTableDimensions=1  BreakpointsForDimension1="[0  5]"  Table="[tractionControl.Kp_start  tractionControl.Kp_end]*tractionControl.Kp_scaling"  ExtrapMethod=Clip  UseLastTableValue=on  InternalRulePriority=Speed  RndMeth=Simplest  InputSameDT=on
  MATLAB Function : MATLAB Function  TreatAsAtomicUnit=on
  MATLAB Function1 : MATLAB Function  TreatAsAtomicUnit=on
  Slip Rate FL : Subsystem
  Slip Rate FL1 : Subsystem
  Slip Rate FL2 : Subsystem
  Slip Rate FL3 : Subsystem
  Ti_SR : Outport
  wires:
  states/1 -> MATLAB Function1/1(states), Slip Rate FL/4(states), Slip Rate FL1/4(states), Slip Rate FL2/4(states), Slip Rate FL3/4(states), MATLAB Function/9(states)
  Ti_ref/1 -> Bus Selector/1
  Bus Selector/1 -> [Ti_FL]  "<FL>"
  Bus Selector/2 -> [Ti_FR]  "<FR>"
  Bus Selector/3 -> [Ti_RL]  "<RL>"
  Bus Selector/4 -> [Ti_RR]  "<RR>"
  [SR_Kp] -> Slip Rate FL/2(Kp)
  Kp Lookup/1 -> ?
  Ki Loopup/1 -> [SR_Ki]
  Gain/1 -> Kp Lookup/1
  Gain2/1 -> Ki Loopup/1
  Constant1/1 -> ?
  Constant/1 -> [SR_Kp]
  MATLAB Function/1(Ti_lim) -> Ti_SR/1
  [Ti_FL] -> MATLAB Function/1(Ti_FL)
  [Ti_RR] -> MATLAB Function/4(Ti_RR)
  [Ti_RL] -> MATLAB Function/3(Ti_RL)
  [Ti_FR] -> MATLAB Function/2(Ti_FR)
  T_requested/1 -> MATLAB Function/10(T_req)
  MATLAB Function1/1(SR_FL) -> Slip Rate FL/3(SR)
  Constant2/1 -> Slip Rate FL3/1(SR_ref), Slip Rate FL2/1(SR_ref), Slip Rate FL1/1(SR_ref), Slip Rate FL/1(SR_ref)
  MATLAB Function1/5(vx) -> Gain2/1, Gain/1
  MATLAB Function1/2(SR_FR) -> Slip Rate FL1/3(SR)
  MATLAB Function1/3(SR_RL) -> Slip Rate FL2/3(SR)
  MATLAB Function1/4(SR_RR) -> Slip Rate FL3/3(SR)
  [SR_Kp] -> Slip Rate FL1/2(Kp)
  [SR_Kp] -> Slip Rate FL2/2(Kp)
  [SR_Kp] -> Slip Rate FL3/2(Kp)
  Slip Rate FL/1(Tc) -> MATLAB Function/5(TC_FL)
  Slip Rate FL1/1(Tc) -> MATLAB Function/6(TC_FR)
  Slip Rate FL2/1(Tc) -> MATLAB Function/7(TC_RL)
  Slip Rate FL3/1(Tc) -> MATLAB Function/8(TC_RR)

== system TV_2017/CarMaker/Control_System /Slip Rate Control /SUM ==
  note: consider to scale FL&FR for steer angle
  In1 : Inport
  Bus Selector : BusSelector  OutputSignals=FL,FR,RL,RR
  Sum : Sum  Inputs=|++
  Sum1 : Sum  Inputs=|++
  Sum2 : Sum  Inputs=|++
  Out1 : Outport
  wires:
  In1/1 -> Bus Selector/1
  Bus Selector/1 -> Sum/1  "<FL>"
  Bus Selector/2 -> Sum1/1  "<FR>"
  Bus Selector/3 -> Sum2/1  "<RL>"
  Bus Selector/4 -> Sum2/2  "<RR>"
  Sum2/1 -> Sum1/2
  Sum1/1 -> Sum/2
  Sum/1 -> Out1/1

== system TV_2017/CarMaker/Control_System /Slip Rate Control /Traction Controllers ==
  states : Inport
  Ti_ref : Inport  Port=2
  T_requested : Inport  Port=3
  Bus Selector : BusSelector  OutputSignals=FL,FR,RL,RR
  Constant2 : Constant  Value=tractionControl.Slip_ratio_ref
  MATLAB Function : MATLAB Function  TreatAsAtomicUnit=on
  MATLAB Function1 : MATLAB Function  TreatAsAtomicUnit=on
  Mux18 : Mux
  Slip Rate FL : Subsystem
  Slip Rate FR : Subsystem
  Slip Rate RL : Subsystem
  Slip Rate RR : Subsystem
  tcOutput : Scope
  tcOutput1 : Scope  NumInputPorts=4
  Ti_SR : Outport
  wires:
  states/1 -> MATLAB Function1/1(states), MATLAB Function/9(states)
  Ti_ref/1 -> MATLAB Function1/3(T_tv), Bus Selector/1
  Bus Selector/1 -> [Ti_FL]  "<FL>"
  Bus Selector/2 -> [Ti_FR]  "<FR>"
  Bus Selector/3 -> [Ti_RL]  "<RL>"
  Bus Selector/4 -> [Ti_RR]  "<RR>"
  [Ti_FL] -> Slip Rate FL/5(Ti_ref)
  [Ti_FR] -> Slip Rate FR/5(Ti_ref)
  [Ti_RL] -> Slip Rate RL/5(Ti_ref)
  [Ti_RR] -> Slip Rate RR/5(Ti_ref)
  [SR_Ki] -> Slip Rate FL/3(Ki)
  [SR_Kp] -> Slip Rate FL/2(Kp)
  [SR_Kp] -> Slip Rate FR/2(Kp)
  [SR_Ki] -> Slip Rate FR/3(Ki)
  [SR_Kp] -> Slip Rate RL/2(Kp)
  [SR_Ki] -> Slip Rate RL/3(Ki)
  [SR_Kp] -> Slip Rate RR/2(Kp)
  [SR_Ki] -> Slip Rate RR/3(Ki)
  Slip Rate FL/1(TC_output) -> Mux18/1, MATLAB Function/5(TC_FL)  "FL"
  Slip Rate FR/1(TC_output) -> Mux18/2, MATLAB Function/6(TC_FR)  "FR"
  Slip Rate RR/1(TC_output) -> Mux18/4, MATLAB Function/8(TC_RR)  "RR"
  Slip Rate RL/1(TC_output) -> Mux18/3, MATLAB Function/7(TC_RL)  "RL"
  MATLAB Function/1(Ti_lim) -> Ti_SR/1
  [Ti_FL] -> MATLAB Function/1(Ti_FL)
  [Ti_RR] -> MATLAB Function/4(Ti_RR)
  [Ti_RL] -> MATLAB Function/3(Ti_RL)
  [Ti_FR] -> MATLAB Function/2(Ti_FR)
  T_requested/1 -> MATLAB Function1/2(T_req), MATLAB Function/10(T_req)
  MATLAB Function1/2(SR_FR) -> tcOutput1/2, Slip Rate FR/4(SR)
  MATLAB Function1/3(SR_RL) -> tcOutput1/3, Slip Rate RL/4(SR)
  Constant2/1 -> Slip Rate RL/1(SR_ref), Slip Rate FR/1(SR_ref), Slip Rate FL/1(SR_ref), Slip Rate RR/1(SR_ref)
  MATLAB Function1/1(SR_FL) -> tcOutput1/1, Slip Rate FL/4(SR)
  MATLAB Function1/5(Kp) -> [SR_Kp]
  MATLAB Function1/6(Ki) -> [SR_Ki]
  Mux18/1 -> tcOutput/1
  MATLAB Function1/4(SR_RR) -> tcOutput1/4, Slip Rate RR/4(SR)

== system TV_2017/CarMaker/Control_System /Subsystem/2016 adapted ==
  note: This needs more thought
  Mz_ref : Inport
  T_req : Inport  Port=2
  "States " : Inport  Port=3
  Bus Selector : BusSelector  OutputSignals=mmt_FL,mmt_FR,mmt_RL,mmt_RR
  Constant{1..4} (4 alike) : Constant  Value=int8(0)
  Inverter temperature limiter : MATLAB Function  TreatAsAtomicUnit=on
  MATLAB Function : MATLAB Function  Commented=on  TreatAsAtomicUnit=on
  Motor temperature limiter : MATLAB Function  TreatAsAtomicUnit=on
  Mux18 : Mux
  Mux2 : Mux
  Torque Allocation : Subsystem
  "max combined tire torque based on (Fz, SA,mu) " : MATLAB Function  TreatAsAtomicUnit=on
  "max long tire torque based on (FZ , mu)" : MATLAB Function  TreatAsAtomicUnit=on
  "max torque " : MATLAB Function  TreatAsAtomicUnit=on
  maxMotorTorque and kers based on available power : MATLAB Function  TreatAsAtomicUnit=on
  maxmotortoruq : Scope
  "Mz_allocated " : Outport
  Ti_lim : Outport  Port=2
  saturated_constraints : Outport  Port=3
  Max_motor_torque : Outport  Port=4
  active_constraints : Outport  Port=5
  wires:
  "States "/1 -> [states], Torque Allocation/2(states)
  Mz_ref/1 -> Torque Allocation/4(Mz_ref)
  Bus Selector/1 -> Mux18/1  "<mmt_FL>"
  Bus Selector/2 -> Mux18/2  "<mmt_FR>"
  Bus Selector/3 -> Mux18/3  "<mmt_RL>"
  Bus Selector/4 -> Mux18/4  "<mmt_RR>"
  T_req/1 -> Torque Allocation/1(T_req)
  Torque Allocation/1(Ti_lim) -> Ti_lim/1
  Mux18/1 -> maxmotortoruq/1
  [states] -> maxMotorTorque and kers based on available power/1(states)
  Inverter temperature limiter/1(maxMotorTorque) -> "max torque "/1(calc_pow_lim), "max torque "/2(inv_temp_lim)
  "max torque "/1(maxMotorTorque) -> Max_motor_torque/1, Bus Selector/1, [maxMotorTorque]
  "max torque "/2(active_constraints) -> active_constraints/1, [active_constraints]
  [states] -> Inverter temperature limiter/1(states)
  Motor temperature limiter/1(maxMotorTorque) -> "max torque "/3(mot_temp_lim)
  [states] -> Motor temperature limiter/1(states)
  "max long tire torque based on (FZ , mu)"/1(maxMotorTorque) -> "max torque "/5(SA_lim), "max torque "/4(mu_lim)
  [states] -> "max long tire torque based on (FZ , mu)"/1(states)
  "max combined tire torque based on (Fz, SA,mu) "/1(maxMotorTorque) -> ?
  [states] -> "max combined tire torque based on (Fz, SA,mu) "/1(states)
  maxMotorTorque and kers based on available power/1(maxMotorTorque) -> ?
  Mux2/1 -> saturated_constraints/1
  Constant1/1 -> Mux2/1  "<mmt_FL>"
  Constant2/1 -> Mux2/2  "<mmt_FR>"
  Constant3/1 -> Mux2/3  "<mmt_RL>"
  Constant4/1 -> Mux2/4  "<mmt_RR>"
  Torque Allocation/2(Mz_allocated) -> "Mz_allocated "/1
  [maxMotorTorque] -> Torque Allocation/3(maxMotorTorque)

== system TV_2017/CarMaker/Control_System /Subsystem/Torque allocation 2016 ==
  Mz_ref : Inport
  T_req : Inport  Port=2
  "States " : Inport  Port=3
  Bus Selector : BusSelector  OutputSignals=mmt_FL,mmt_FR,mmt_RL,mmt_RR
  MATLAB Function : MATLAB Function  TreatAsAtomicUnit=on
  Mux18 : Mux
  Torque Allocation : Subsystem
  maxmotortoruq : Scope
  Ti_lim : Outport
  "Mz_error " : Outport  Port=2
  Max_motor_torque_i : Outport  Port=3
  wires:
  "States "/1 -> MATLAB Function/1(states), Torque Allocation/2(states)
  Mz_ref/1 -> Torque Allocation/4(Mz_ref)
  Torque Allocation/2(Mz_error) -> "Mz_error "/1
  MATLAB Function/1(maxMotorTorque) -> Bus Selector/1, Torque Allocation/3(maxMotorTorque)
  Bus Selector/1 -> Mux18/1  "<mmt_FL>"
  Bus Selector/2 -> Mux18/2  "<mmt_FR>"
  Bus Selector/3 -> Mux18/3  "<mmt_RL>"
  Bus Selector/4 -> Mux18/4  "<mmt_RR>"
  T_req/1 -> Torque Allocation/1(T_req)
  Torque Allocation/1(Ti_lim) -> Ti_lim/1
  Mux18/1 -> Max_motor_torque_i/1, maxmotortoruq/1

== system TV_2017/CarMaker/Control_System /Subsystem/Torque allocation 2017 ==
  Mz_ref : Inport
  T_req : Inport  Port=2
  "States " : Inport  Port=3
  Bus Creator : BusCreator  Commented=on  Inputs=2  OutDataTypeStr=Bus: maxMotorTorque
  Bus Selector1 : BusSelector  Commented=on  OutputSignals=mmt_FL,mmt_FR,mmt_RL,mmt_RR
  Constant{1..4} (4 alike) : Constant  Value=int8(1)
  Inverter temperature limiter : MATLAB Function  TreatAsAtomicUnit=on
  Motor temperature limiter : MATLAB Function  TreatAsAtomicUnit=on
  Mux2 : Mux
  Scope : Scope
  Scope1 : Scope  Commented=on  NumInputPorts=4
  Torque Allocation Quadratic Programming : MATLAB Function  TreatAsAtomicUnit=on
  "max combined tire torque based on (Fz, SA,mu) " : MATLAB Function  TreatAsAtomicUnit=on
  "max long tire torque based on (FZ , mu)" : MATLAB Function  TreatAsAtomicUnit=on
  "max torque " : MATLAB Function  TreatAsAtomicUnit=on
  maxMotorTorque and kers based on available power : MATLAB Function  TreatAsAtomicUnit=on
  "Mz_allocated " : Outport
  Ti_lim : Outport  Port=2
  saturated_constraints : Outport  Port=3
  max_motor_torque : Outport  Port=4
  active_constraints : Outport  Port=5
  wires:
  [states] -> maxMotorTorque and kers based on available power/1(states)
  "max torque "/2(active_constraints) -> [active_constraints]
  [states] -> Inverter temperature limiter/1(states)
  Motor temperature limiter/1(maxMotorTorque) -> "max torque "/4(mot_temp_lim)
  [states] -> Motor temperature limiter/1(states)
  "max long tire torque based on (FZ , mu)"/1(maxMotorTorque) -> "max torque "/2(SA_lim), "max torque "/1(mu_lim)
  [states] -> "max long tire torque based on (FZ , mu)"/1(states)
  [states] -> "max combined tire torque based on (Fz, SA,mu) "/1(states)
  [maxMotorTorque] -> max_motor_torque/1
  [active_constraints] -> active_constraints/1
  Mux2/1 -> saturated_constraints/1
  Constant1/1 -> Mux2/1  "<mmt_FL>"
  Constant2/1 -> Mux2/2  "<mmt_FR>"
  Constant3/1 -> Mux2/3  "<mmt_RL>"
  Constant4/1 -> Mux2/4  "<mmt_RR>"
  Mz_ref/1 -> ?  "Mz_ref"
  T_req/1 -> ?
  "States "/1 -> [states]
  [states] -> ?
  [maxMotorTorque] -> ?
  ? -> Ti_lim/1
  ? -> "Mz_allocated "/1
  "max torque "/1(maxMotorTorque) -> Bus Selector1/1, [maxMotorTorque]
  Bus Selector1/1 -> Scope1/1  "<mmt_FL>"
  Bus Selector1/2 -> Scope1/2  "<mmt_FR>"
  Bus Selector1/3 -> Scope1/3  "<mmt_RL>"
  Bus Selector1/4 -> Scope1/4  "<mmt_RR>"
  Inverter temperature limiter/1(maxMotorTorque) -> "max torque "/3(inv_temp_lim)
  "max combined tire torque based on (Fz, SA,mu) "/1(maxMotorTorque) -> ?

== system TV_2017/CarMaker/Control_System /Subsystem/Torque allocation QP- ==
  Mz_ref : Inport
  T_req : Inport  Port=2
  "States " : Inport  Port=3
  Bus Creator : BusCreator  Commented=on  Inputs=2  OutDataTypeStr=Bus: maxMotorTorque
  Bus Selector1 : BusSelector  OutputSignals=mmt_FL,mmt_FR,mmt_RL,mmt_RR
  Constant{1..4} (4 alike) : Constant  Value=int8(1)
  Inverter temperature limiter : MATLAB Function  TreatAsAtomicUnit=on
  Motor temperature limiter : MATLAB Function  TreatAsAtomicUnit=on
  Mux2 : Mux
  Scope : Scope
  Scope1 : Scope  NumInputPorts=4
  Torque Allocation Quadratic Programming : MATLAB Function  TreatAsAtomicUnit=on
  "max combined tire torque based on (Fz, SA,mu) " : MATLAB Function  TreatAsAtomicUnit=on
  "max long tire torque based on (FZ , mu)" : MATLAB Function  TreatAsAtomicUnit=on
  "max torque " : MATLAB Function  TreatAsAtomicUnit=on
  maxMotorTorque and kers based on available power : MATLAB Function  TreatAsAtomicUnit=on
  "Mz_allocated " : Outport
  Ti_lim : Outport  Port=2
  saturated_constraints : Outport  Port=3
  max_motor_torque : Outport  Port=4
  active_constraints : Outport  Port=5
  wires:
  [states] -> maxMotorTorque and kers based on available power/1(states)
  "max torque "/2(active_constraints) -> [active_constraints]
  [states] -> Inverter temperature limiter/1(states)
  Motor temperature limiter/1(maxMotorTorque) -> "max torque "/4(mot_temp_lim)
  [states] -> Motor temperature limiter/1(states)
  "max long tire torque based on (FZ , mu)"/1(maxMotorTorque) -> "max torque "/2(SA_lim), "max torque "/1(mu_lim)
  [states] -> "max long tire torque based on (FZ , mu)"/1(states)
  [states] -> "max combined tire torque based on (Fz, SA,mu) "/1(states)
  [maxMotorTorque] -> max_motor_torque/1
  [active_constraints] -> active_constraints/1
  Mux2/1 -> saturated_constraints/1
  Constant1/1 -> Mux2/1  "<mmt_FL>"
  Constant2/1 -> Mux2/2  "<mmt_FR>"
  Constant3/1 -> Mux2/3  "<mmt_RL>"
  Constant4/1 -> Mux2/4  "<mmt_RR>"
  Mz_ref/1 -> Torque Allocation Quadratic Programming/1(Mz_ref)  "Mz_ref"
  T_req/1 -> Torque Allocation Quadratic Programming/2(T_req)
  "States "/1 -> [states]
  [states] -> Torque Allocation Quadratic Programming/3(states)
  [maxMotorTorque] -> Torque Allocation Quadratic Programming/4(maxMotorTorque)
  Torque Allocation Quadratic Programming/1(Ti_lim) -> Ti_lim/1
  Torque Allocation Quadratic Programming/3(Mz_allocated) -> "Mz_allocated "/1
  "max torque "/1(maxMotorTorque) -> Bus Selector1/1, [maxMotorTorque]
  Bus Selector1/1 -> Scope1/1  "<mmt_FL>"
  Bus Selector1/2 -> Scope1/2  "<mmt_FR>"
  Bus Selector1/3 -> Scope1/3  "<mmt_RL>"
  Bus Selector1/4 -> Scope1/4  "<mmt_RR>"
  Inverter temperature limiter/1(maxMotorTorque) -> "max torque "/3(inv_temp_lim)

== system TV_2017/CarMaker/Control_System /Subsystem/Torque allocation QP-1 ==
  Mz_ref : Inport
  T_req : Inport  Port=2
  "States " : Inport  Port=3
  Bus Creator : BusCreator  Commented=on  Inputs=2  OutDataTypeStr=Bus: maxMotorTorque
  Bus Selector1 : BusSelector  OutputSignals=mmt_FL,mmt_FR,mmt_RL,mmt_RR
  Constant{1..4} (4 alike) : Constant  Value=int8(1)
  Inverter temperature limiter : MATLAB Function  TreatAsAtomicUnit=on
  Motor temperature limiter : MATLAB Function  TreatAsAtomicUnit=on
  Mux2 : Mux
  Scope : Scope
  Scope1 : Scope  NumInputPorts=4
  Torque Allocation Quadratic Programming : MATLAB Function  TreatAsAtomicUnit=on
  "max combined tire torque based on (Fz, SA,mu) " : MATLAB Function  TreatAsAtomicUnit=on
  "max long tire torque based on (FZ , mu)" : MATLAB Function  TreatAsAtomicUnit=on
  "max torque " : MATLAB Function  TreatAsAtomicUnit=on
  maxMotorTorque and kers based on available power : MATLAB Function  TreatAsAtomicUnit=on
  "Mz_allocated " : Outport
  Ti_lim : Outport  Port=2
  saturated_constraints : Outport  Port=3
  max_motor_torque : Outport  Port=4
  active_constraints : Outport  Port=5
  wires:
  [states] -> maxMotorTorque and kers based on available power/1(states)
  "max torque "/2(active_constraints) -> [active_constraints]
  [states] -> Inverter temperature limiter/1(states)
  Motor temperature limiter/1(maxMotorTorque) -> "max torque "/4(mot_temp_lim)
  [states] -> Motor temperature limiter/1(states)
  "max long tire torque based on (FZ , mu)"/1(maxMotorTorque) -> "max torque "/2(SA_lim), "max torque "/1(mu_lim)
  [states] -> "max long tire torque based on (FZ , mu)"/1(states)
  [states] -> "max combined tire torque based on (Fz, SA,mu) "/1(states)
  [maxMotorTorque] -> max_motor_torque/1
  [active_constraints] -> active_constraints/1
  Mux2/1 -> saturated_constraints/1
  Constant1/1 -> Mux2/1  "<mmt_FL>"
  Constant2/1 -> Mux2/2  "<mmt_FR>"
  Constant3/1 -> Mux2/3  "<mmt_RL>"
  Constant4/1 -> Mux2/4  "<mmt_RR>"
  Mz_ref/1 -> Torque Allocation Quadratic Programming/1(Mz_ref)  "Mz_ref"
  T_req/1 -> Torque Allocation Quadratic Programming/2(T_req)
  "States "/1 -> [states]
  [states] -> Torque Allocation Quadratic Programming/3(states)
  [maxMotorTorque] -> Torque Allocation Quadratic Programming/4(maxMotorTorque)
  Torque Allocation Quadratic Programming/1(Ti_lim) -> Ti_lim/1
  Torque Allocation Quadratic Programming/3(Mz_allocated) -> "Mz_allocated "/1
  "max torque "/1(maxMotorTorque) -> Bus Selector1/1, [maxMotorTorque]
  Bus Selector1/1 -> Scope1/1  "<mmt_FL>"
  Bus Selector1/2 -> Scope1/2  "<mmt_FR>"
  Bus Selector1/3 -> Scope1/3  "<mmt_RL>"
  Bus Selector1/4 -> Scope1/4  "<mmt_RR>"
  Inverter temperature limiter/1(maxMotorTorque) -> "max torque "/3(inv_temp_lim)

== system TV_2017/CarMaker/Control_System /TA 2017/Slip handling (Traction Control)  ==
  Sensors : Inport
  Memory : Memory  InheritSampleTime=on
  Memory1 : Memory  InheritSampleTime=on
  Scaling factors from slip detection : MATLAB Function  TreatAsAtomicUnit=on
  slipScalingFactors : Outport
  wires:
  Sensors/1 -> Scaling factors from slip detection/1(states)
  Scaling factors from slip detection/2(duration) -> Memory1/1
  Memory/1 -> Scaling factors from slip detection/3(prev_slip)
  Scaling factors from slip detection/3(slip) -> Memory/1
  Memory1/1 -> Scaling factors from slip detection/2(prev_duration)
  Scaling factors from slip detection/1(slipScalingFactor) -> slipScalingFactors/1

== system TV_2017/CarMaker/Control_System /Yaw_rate_Mz_generator/Yaw Rate Controller  ==
  "Mz_error " : Inport
  States : Inport  Port=2
  Data Type Conversion : DataTypeConversion  OutDataTypeStr=single  RndMeth=Round
  Discrete-Time Integrator2 : DiscreteIntegrator  InitialConditionSetting=State (most efficient)  SampleTime=-1  LimitOutput=on  UpperSaturationLimit=yawRateControl.max_moment  LowerSaturationLimit=-yawRateControl.max_moment  ICPrevOutput=DiscIntNeverNeededParam  ICPrevScaledInput=DiscIntNeverNeededParam
  Enable/disable : Constant  Value=yawRateControl.enable
  Gain1 : Gain  Gain=single(3.6)
  Ksat : Constant  Value=yawRateControl.Ksat
  Memory : Memory  InheritSampleTime=on
  Mz_ref_YRR : Scope  NumInputPorts=2
  "Mzerror " : Scope
  Mzerror 1 : Scope  NumInputPorts=2
  PI_Ki 3 : Scope
  Product{7..8,10..11} (4 alike) : Product
  Product3 : Product  OutDataTypeStr=single
  Saturation : Saturate  UpperLimit=yawRateControl.max_moment  LowerLimit=-yawRateControl.max_moment
  Sum2 : Sum  Inputs=+++  AccumDataTypeStr=single
  Sum3 : Sum  Inputs=|+-
  gainScheduling : MATLAB Function  TreatAsAtomicUnit=on
  "not NaN " : MATLAB Function  TreatAsAtomicUnit=on
  not not a number : MATLAB Function  TreatAsAtomicUnit=on
  yawRateReference : MATLAB Function  TreatAsAtomicUnit=on
  "r_ref " : Outport
  r_lim : Outport  Port=2
  Mz_ref : Outport  Port=3  OutDataTypeStr=single
  Mz_ref_to_telemetry : Outport  Port=4  OutDataTypeStr=single
  wires:
  States/1 -> yawRateReference/1(states)
  yawRateReference/4(r_ref) -> "r_ref "/1
  yawRateReference/5(r_lim) -> r_lim/1
  Product7/1 -> Sum2/2
  Sum2/1 -> Mz_ref_to_telemetry/1, Product3/2
  Product8/1 -> Sum3/1
  Sum3/1 -> Discrete-Time Integrator2/1
  Discrete-Time Integrator2/1 -> PI_Ki 3/1, Sum2/3
  Product11/1 -> not not a number/1(in)
  yawRateReference/1(r_der_error) -> Product10/1
  Product10/1 -> Sum2/1
  gainScheduling/2(Kp) -> Mzerror 1/1, Product7/1
  Ksat/1 -> Product11/1
  "Mz_error "/1 -> "Mzerror "/1, Product11/2
  gainScheduling/3(Ki) -> Product8/1, Mzerror 1/2
  yawRateReference/2(r_error) -> Memory/1, Product8/2, Product7/2
  Product3/1 -> Saturation/1
  Enable/disable/1 -> Product3/1
  yawRateReference/3(vx) -> Gain1/1
  Gain1/1 -> gainScheduling/1(vx_kmh)
  gainScheduling/1(Kd) -> Product10/2
  not not a number/1(out) -> Sum3/2
  Saturation/1 -> "not NaN "/1(in)
  "not NaN "/1(out) -> Data Type Conversion/1, Mz_ref_YRR/1
  Data Type Conversion/1 -> Mz_ref_YRR/2, Mz_ref/1
  Memory/1 -> yawRateReference/2(prev_r_error)

== system TV_2017/CarMaker/Control_System /Yaw_rate_Mz_generator/Yaw Rate Generator ==
  States : Inport
  Yaw Rate ref : Scope  NumInputPorts=3
  yawRateGenerator : MATLAB Function  TreatAsAtomicUnit=on
  Mz_ref : Outport  OutDataTypeStr=single
  Mz_ref_to_telemetry : Outport  Port=2  OutDataTypeStr=single
  wires:
  yawRateGenerator/1(Mz_ref) -> Yaw Rate ref/1, Mz_ref/1
  States/1 -> yawRateGenerator/1(states)
  yawRateGenerator/3(Kp_term) -> Yaw Rate ref/2
  yawRateGenerator/4(Kd_term) -> Yaw Rate ref/3
  yawRateGenerator/2(Mz_ref_to_telemetry) -> Mz_ref_to_telemetry/1
